simulink model "THI"  (R2023a)
settings: Solver=ode23tb  StartTime=0.0  StopTime=.1  MaxStep=1e-4  RelTol=1e-3
libraries: spsMosfetLib x6, simulink x3, spsDCVoltageSourceLib x1, spsGroundLib x1, spsThreePhaseSeriesRLCBranchLib x1, spsThreePhaseVIMeasurementLib x1, sps_lib x1
settings Model: Creator=gaming3  LastModifiedBy=gaming3

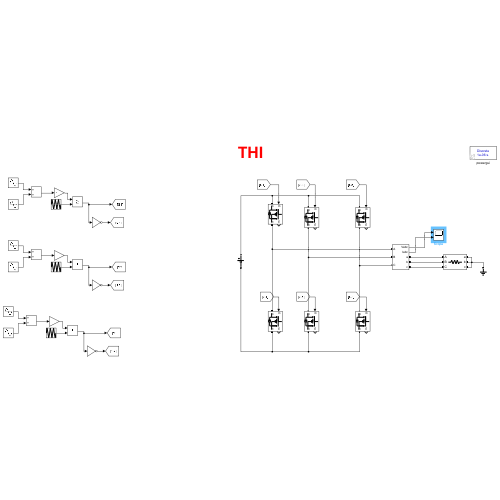
[thumbnail: Simulink's stored preview of the top-level diagram]
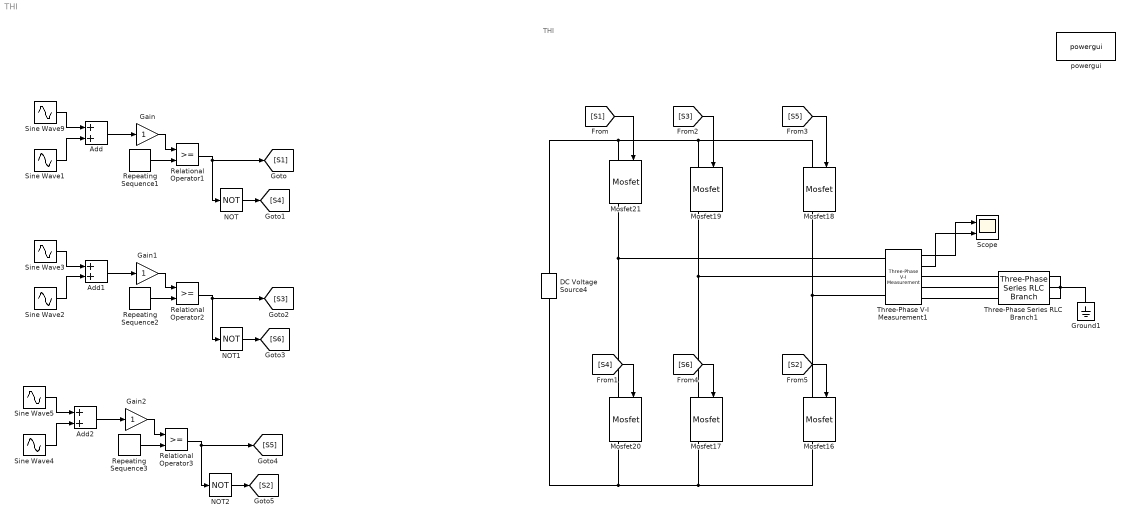
== system THI ==
  note: THI
  Add : Sum
  Add1 : Sum
  Add2 : Sum
  DC Voltage Source4 : spsDCVoltageSourceLib/DC Voltage Source  Amplitude=310  Measurements=None
  Gain : Gain
  Gain1 : Gain
  Gain2 : Gain
  Ground1 : spsGroundLib/Ground  LConnTagsString=a
  Mosfet{16..21} (6 alike) : spsMosfetLib/Mosfet  Ron=0.1  Lon=0  Rd=0.01  Vfd=0  IC=0  Rs=1e5  Cs=inf  Measurements=on
  NOT : Logic  Operator=NOT  IconShape=distinctive  AllPortsSameDT=off  OutDataTypeStr=boolean
  NOT1 : Logic  Operator=NOT  IconShape=distinctive  AllPortsSameDT=off  OutDataTypeStr=boolean
  NOT2 : Logic  Operator=NOT  IconShape=distinctive  AllPortsSameDT=off  OutDataTypeStr=boolean
  Relational Operator1 : RelationalOperator  OutDataTypeStr=boolean  RndMeth=Simplest  InputSameDT=off
  Relational Operator2 : RelationalOperator  OutDataTypeStr=boolean  RndMeth=Simplest  InputSameDT=off
  Relational Operator3 : RelationalOperator  OutDataTypeStr=boolean  RndMeth=Simplest  InputSameDT=off
  Repeating Sequence1 : simulink/Sources/Repeating Sequence  rep_seq_t=[0 (1/5000)/4 (1/5000)/2 (3/5000)/4 (1/5000)]  rep_seq_y=[0 1 0 -1 0]
  Repeating Sequence2 : simulink/Sources/Repeating Sequence  rep_seq_t=[0 (1/5000)/4 (1/5000)/2 (3/5000)/4 (1/5000)]  rep_seq_y=[0 1 0 -1 0]
  Repeating Sequence3 : simulink/Sources/Repeating Sequence  rep_seq_t=[0 (1/5000)/4 (1/5000)/2 (3/5000)/4 (1/5000)]  rep_seq_y=[0 1 0 -1 0]
  Scope : Scope  NumInputPorts=2
  Sine Wave1 : Sin  Amplitude=0.19  Frequency=300*pi  SampleTime=0
  Sine Wave2 : Sin  Amplitude=0.19  Frequency=300*pi  SampleTime=0
  Sine Wave3 : Sin  Amplitude=1.15  Frequency=100*pi  Phase=-(2*pi)/3  SampleTime=0
  Sine Wave4 : Sin  Amplitude=0.19  Frequency=300*pi  SampleTime=0
  Sine Wave5 : Sin  Amplitude=1.15  Frequency=100*pi  Phase=(2*pi)/3  SampleTime=0
  Sine Wave9 : Sin  Amplitude=1.15  Frequency=100*pi  SampleTime=0
  Three-Phase Series RLC Branch1 : spsThreePhaseSeriesRLCBranchLib/Three-Phase Series RLC Branch  LConnTagsString=A|B|C  RConnTagsString=A|B|C  BranchType=R  Resistance=10  Inductance=1e-3  Capacitance=1e-6  Measurements=None
  Three-Phase V-I Measurement1 : spsThreePhaseVIMeasurementLib/Three-Phase V-I Measurement  VoltageMeasurement=phase-to-ground  SetLabelV=off  LabelV=Vabc  Vpu=off  VpuLL=off  CurrentMeasurement=yes  SetLabelI=off  LabelI=Iabc  Ipu=off  Pbase=100e6  Vbase=500e3  OutputType=Complex  PhasorSimulation=off  PSBequivalent=0
  powergui : sps_lib/powergui  Priority=1  SimulationMode=Discrete  SampleTime=1e-06  frequency=60  Iterations=50  frequencyindice=0  Pbase=100e6  ErrMax=1e-4  UnitsV=kV  UnitsW=MW  buscounter=0  FunctionMessages=off  echomessages=off  EnableUseOfTLC=off  CurrentSourceSwitches=off  DisableSnubberDevices=off  DisableRonSwitches=off  DisableVfSwitches=off  DisplayEquations=off  AutomaticDiscreteSolvers=off  SolverType=Tustin/Backward Euler (TBE)  Interpol=off  ExternalGateDelay=off  methode=off  Ts=100  x0status=blocks  SPID=on  SwTol=0  HookPort=off  NonlinearTolerance=1e-4  nMaxIteration=100  ContinueOnMaxIteration=off  RestoreLinks=warning  ResistiveCurrentMeasurement=off  Frange=[0:2:500]  Ylog=off  Xlog=on  ShowGrid=off  save=off  variable=ZData  structure=0  ZoomFFT=off  StartTime=0.0  cycles=1  DisplayStyle=1  fundamental=60  FreqAxis=off  MaxFrequency=1000  frequencyindicesteady=1  RmsSteady=1  display=off
  wires:
  Sine Wave9/1 -> Add/1
  Sine Wave1/1 -> Add/2
  Repeating Sequence1/1 -> Relational Operator1/2
  Add/1 -> Gain/1
  Gain/1 -> Relational Operator1/1
  [S2] -> Mosfet16/1
  [S5] -> Mosfet18/1
  [S6] -> Mosfet17/1
  [S3] -> Mosfet19/1
  [S4] -> Mosfet20/1
  [S1] -> Mosfet21/1
  Relational Operator1/1 -> NOT/1, [S1]
  NOT/1 -> [S4]
  NOT1/1 -> [S6]
  Relational Operator2/1 -> [S3], NOT1/1
  Gain1/1 -> Relational Operator2/1
  Add1/1 -> Gain1/1
  Repeating Sequence2/1 -> Relational Operator2/2
  Sine Wave2/1 -> Add1/2
  Sine Wave3/1 -> Add1/1
  Sine Wave5/1 -> Add2/1
  Sine Wave4/1 -> Add2/2
  Repeating Sequence3/1 -> Relational Operator3/2
  Add2/1 -> Gain2/1
  Gain2/1 -> Relational Operator3/1
  Relational Operator3/1 -> NOT2/1, [S5]
  NOT2/1 -> [S2]
  Three-Phase V-I Measurement1/1 -> Scope/1
  Three-Phase V-I Measurement1/2 -> Scope/2
  connections:
  Three-Phase Series RLC Branch1/RConn1 -- Ground1/LConn1 -- Three-Phase Series RLC Branch1/RConn2 -- Three-Phase Series RLC Branch1/RConn3
  DC Voltage Source4/LConn1 -- Mosfet17/RConn1 -- Mosfet16/RConn1 -- Mosfet20/RConn1
  Mosfet18/LConn1 -- Mosfet19/LConn1 -- DC Voltage Source4/RConn1 -- Mosfet21/LConn1
  Mosfet17/LConn1 -- Mosfet19/RConn1 -- Three-Phase V-I Measurement1/LConn2
  Three-Phase V-I Measurement1/LConn1 -- Mosfet21/RConn1 -- Mosfet20/LConn1
  Mosfet16/LConn1 -- Mosfet18/RConn1 -- Three-Phase V-I Measurement1/LConn3
  Three-Phase Series RLC Branch1/LConn1 -- Three-Phase V-I Measurement1/RConn1
  Three-Phase Series RLC Branch1/LConn2 -- Three-Phase V-I Measurement1/RConn2
  Three-Phase Series RLC Branch1/LConn3 -- Three-Phase V-I Measurement1/RConn3
